simulink model "boh"  (R2022b)
settings: Solver=VariableStepAuto  StartTime=0.0  StopTime=10.0  RelTol=1e-3
values from neighbouring files (symbols this model uses):
  I = 5.7    [init.m]
  l = 1    [init.m]
  nr = 5    [init.m]
  theta_0 = 0    [init.m]
  theta_0_dot = 0    [init.m]
  U_0 = m*g_0*d    (= 8.9271)    [init.m]
  viscous = bl + bm*nr^2    (= 53)    [init.m]
settings Model: Creator=Omar Bayoumi  LastModifiedBy=Omar Bayoumi

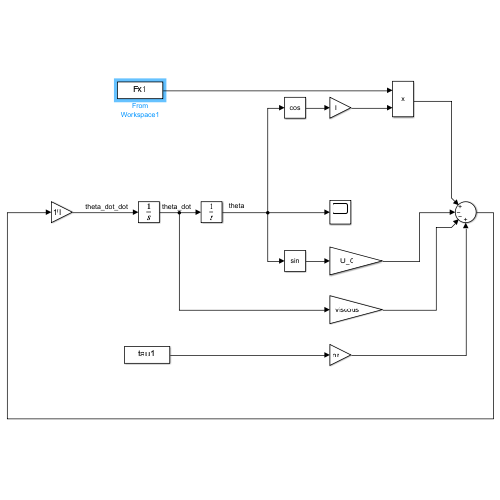
[thumbnail: Simulink's stored preview of the top-level diagram]
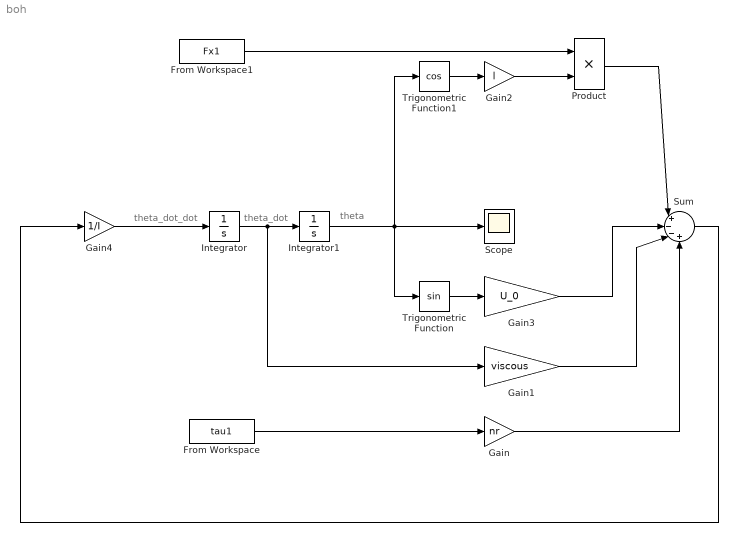
== system boh ==
  note: theta
  note: theta_dot
  note: theta_dot_dot
  From Workspace : FromWorkspace  VariableName=tau1
  From Workspace1 : FromWorkspace  VariableName=Fx1
  Gain : Gain  Gain=nr
  Gain1 : Gain  Gain=viscous
  Gain2 : Gain  Gain=l
  Gain3 : Gain  Gain=U_0
  Gain4 : Gain  Gain=1/I
  Integrator : Integrator  InitialCondition=theta_0_dot
  Integrator1 : Integrator  InitialCondition=theta_0
  Product : Product
  Scope : Scope
  Sum : Sum  Inputs=|+--+
  Trigonometric Function : Trigonometry
  Trigonometric Function1 : Trigonometry  Operator=cos
  wires:
  Integrator/1 -> Gain1/1, Integrator1/1
  Integrator1/1 -> Trigonometric Function/1, Scope/1, Trigonometric Function1/1
  Trigonometric Function/1 -> Gain3/1
  Gain4/1 -> Integrator/1
  Trigonometric Function1/1 -> Gain2/1
  From Workspace1/1 -> Product/1
  Gain2/1 -> Product/2
  Product/1 -> Sum/1
  Gain1/1 -> Sum/3
  Gain3/1 -> Sum/2
  Gain/1 -> Sum/4
  Sum/1 -> Gain4/1
  From Workspace/1 -> Gain/1
